simulink model "flare"  (Simulink 7.5)
settings: Solver=ode45  StartTime=0.0  StopTime=10.0  RelTol=1e-3
undefined symbols (not defined in the file or in its folder): alpha1F, alpha2F, alpha3F, Ap, Bp, cpf, GAMMA, K1F, K2F, T2
settings Model: Creator=ex08148  LastModifiedBy=ex08148

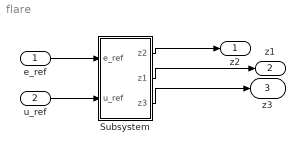
== system flare ==
  e_ref : Inport  OutDataType=sfix(16)  OutScaling=2^0
  u_ref : Inport  Port=2  OutDataType=sfix(16)  OutScaling=2^0
  Subsystem : Subsystem
  z2 : Outport  OutDataType=sfix(16)  OutScaling=2^0
  z1 : Outport  Port=2  OutDataType=sfix(16)  OutScaling=2^0
  z3 : Outport  Port=3  OutDataType=sfix(16)  OutScaling=2^0
  wires:
  Subsystem/1(z2) -> z2/1
  Subsystem/2(z1) -> z1/1
  Subsystem/3(z3) -> z3/1
  e_ref/1 -> Subsystem/1(e_ref)
  u_ref/1 -> Subsystem/2(u_ref)

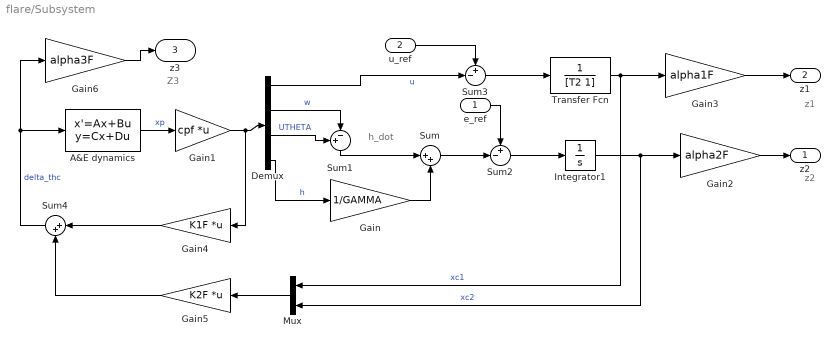
== system flare/Subsystem ==
  note: z2
  note: z1
  note: Z3
  note: h_dot
  e_ref : Inport  OutDataType=sfix(16)  OutScaling=2^0
  u_ref : Inport  Port=2  OutDataType=sfix(16)  OutScaling=2^0
  A&E dynamics : StateSpace  A=Ap  B=Bp
  Demux : Demux
  Gain : Gain  Gain=1/GAMMA  ParameterDataType=sfix(16)  ParameterScaling=2^0  OutDataType=sfix(16)  OutScaling=2^0
  Gain1 : Gain  Gain=cpf  Multiplication=Matrix(K*u)  ParameterDataType=sfix(16)  ParameterScaling=2^0  OutDataType=sfix(16)  OutScaling=2^0
  Gain2 : Gain  Gain=alpha2F  ParameterDataType=sfix(16)  ParameterScaling=2^0  OutDataType=sfix(16)  OutScaling=2^0
  Gain3 : Gain  Gain=alpha1F  ParameterDataType=sfix(16)  ParameterScaling=2^0  OutDataType=sfix(16)  OutScaling=2^0
  Gain4 : Gain  Gain=K1F  Multiplication=Matrix(K*u)  ParameterDataType=sfix(16)  ParameterScaling=2^0  OutDataType=sfix(16)  OutScaling=2^0
  Gain5 : Gain  Gain=K2F  Multiplication=Matrix(K*u)  ParameterDataType=sfix(16)  ParameterScaling=2^0  OutDataType=sfix(16)  OutScaling=2^0
  Gain6 : Gain  Gain=alpha3F  ParameterDataType=sfix(16)  ParameterScaling=2^0  OutDataType=sfix(16)  OutScaling=2^0
  Integrator1 : Integrator
  Mux : Mux  Inputs=2
  Sum : Sum  Inputs=|++  OutDataType=sfix(16)  OutScaling=2^0
  Sum1 : Sum  Inputs=+-|  OutDataType=sfix(16)  OutScaling=2^0
  Sum2 : Sum  Inputs=+-|  OutDataType=sfix(16)  OutScaling=2^0
  Sum3 : Sum  Inputs=+-|  OutDataType=sfix(16)  OutScaling=2^0
  Sum4 : Sum  Inputs=|++  OutDataType=sfix(16)  OutScaling=2^0
  Transfer Fcn : TransferFcn  Denominator=[T2 1]
  z2 : Outport  OutDataType=sfix(16)  OutScaling=2^0
  z1 : Outport  Port=2  OutDataType=sfix(16)  OutScaling=2^0
  z3 : Outport  Port=3  OutDataType=sfix(16)  OutScaling=2^0
  wires:
  A&E dynamics/1 -> Gain1/1  "xp"
  Gain1/1 -> Demux/1, Gain4/1
  Demux/3 -> Sum1/1  "UTHETA"
  Demux/2 -> Sum1/2  "w"
  Demux/4 -> Gain/1  "h"
  Sum1/1 -> Sum/1
  Gain/1 -> Sum/2
  Sum/1 -> Sum2/2
  e_ref/1 -> Sum2/1
  Sum2/1 -> Integrator1/1
  Demux/1 -> Sum3/2  "u"
  u_ref/1 -> Sum3/1
  Sum3/1 -> Transfer Fcn/1
  Integrator1/1 -> Gain2/1, Mux/2  "xc2"
  Gain2/1 -> z2/1
  Transfer Fcn/1 -> Gain3/1, Mux/1  "xc1"
  Gain3/1 -> z1/1
  Mux/1 -> Gain5/1
  Gain5/1 -> Sum4/2
  Gain4/1 -> Sum4/1
  Sum4/1 -> Gain6/1, A&E dynamics/1  "delta_thc"
  Gain6/1 -> z3/1
